simulink model "model_4_3_offset"  (R2020a)
settings: Solver=FixedStepAuto  StartTime=0.0  StopTime=10.0  FixedStep=0.002  RelTol=1e-3
settings Model: Creator=gianlu  LastModifiedBy=Shadman

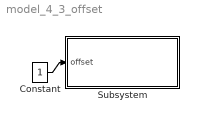
== system model_4_3_offset ==
  Constant : Constant
  Subsystem : Subsystem  StopFcn=|
      | % Cart dimensions
      | x_size = 0.2;
      | y_size = 0.05;
      | wheel_radius = 0.025
      | wheel_pos = 0.08
      | %%
      | % Cart body
      | x = [ - x_size, x_size, x_size, -x_size];
      | y = [ - y_size, -y_size, y_size, y_size];
      | 
      | %%
      | g = hgtransform;
      | %%
      | patch('XData',x,'YData',y,'FaceColor','red','Parent',g)
      | 
      | % Left wheel
      | theta = linspace(0, 2*pi, 15);
      | l_x = - wheel_pos + wheel_radius * cos(theta);
      | l_y = -(y_size + wheel_radius) + wheel_radius * sin(theta);
      | l = hgtransform;
      | patch('XData',l_x,'YData',l_y,'FaceColor','black','Parent', l)
      | 
      | 
      | % Right wheel
      | r_x = wheel_pos + wheel_radius*cos(theta);
      | r_y = -(y_size + wheel_radius) + wheel_radius*sin(theta);
      | r = hgtransform;
      | patch('XData',r_x,'YData',r_y,'FaceColor','black','Parent', r)
      | 
      | 
      | % Plot settings
      | axis equal
      | title('Cart animation')
      | set(gca,'YColor','none')
      | 
      | xlim([-1.5 1.5])
      | ylim([-(y_size+2*wheel_radius), 3 * y_size])
      | set(gca, 'Ytick', [])
      | pt1 = [0 0 0];
      | pt2 = [3 0 0];
      | %%
      | data_pos = out.sim_data_cart.signals.values(:,1);
      | tot_time_step=size(out.tout)/10;
      | 
      | %%
      | for i=1:1:tot_time_step(1)
      |   transf = makehgtform('translate', [1 0 0] * data_pos(i*5));
      |   set(g, 'Matrix', transf);
      |   set(l, 'Matrix', transf);
      |   set(r, 'Matrix', transf);
      | 
      |   %g.Matrix = makehgtform('translate', [1 0 0] * data_pos(i));
      |   %l.Matrix = makehgtform('translate', [1 0 0] * data_pos(i));
      |   %right.Matrix = makehgtform('translate', [1 0 0] * data_pos(i));
      |   %drawnow limitrate
      |   pause(0.02)
      | end
  wires:
  Constant/1 -> Subsystem/1("offset ")

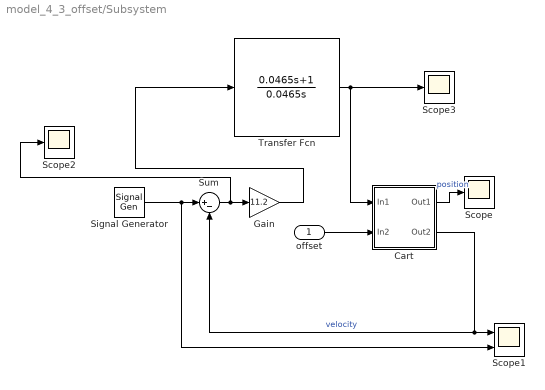
== system model_4_3_offset/Subsystem ==
  "offset " : Inport
  "Cart " : Subsystem  TreatAsAtomicUnit=on
  Gain : Gain  Gain=11.2
  Scope : Scope
  Scope1 : Scope  NumInputPorts=2
  Scope2 : Scope
  Scope3 : Scope
  Signal Generator : SignalGenerator  WaveForm=square  Amplitude=0.2  Frequency=0.5
  Sum : Sum  Inputs=|+-
  Transfer Fcn : TransferFcn  Numerator=[0.0465 1]  Denominator=[0.0465 0]
  wires:
  "offset "/1 -> "Cart "/2(In2)
  "Cart "/1(Out1) -> Scope/1  "position"
  "Cart "/2(Out2) -> Sum/2, Scope1/1  "velocity"
  Signal Generator/1 -> Scope1/2, Sum/1
  Transfer Fcn/1 -> Scope3/1, "Cart "/1(In1)
  Sum/1 -> Scope2/1, Gain/1
  Gain/1 -> Transfer Fcn/1

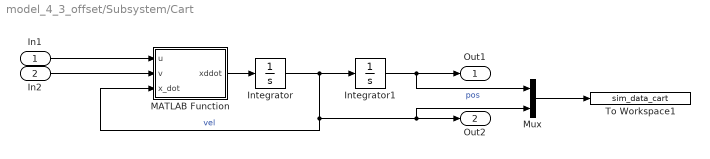
== system model_4_3_offset/Subsystem/Cart  ==
  In1 : Inport
  In2 : Inport  Port=2
  Integrator : Integrator
  Integrator1 : Integrator
  MATLAB Function : MATLAB Function  TreatAsAtomicUnit=on
  Mux : Mux  Inputs=2
  To Workspace1 : ToWorkspace  VariableName=sim_data_cart  SaveFormat=Structure With Time  SampleTime=-1
  Out1 : Outport
  Out2 : Outport  Port=2
  wires:
  MATLAB Function/1(xddot) -> Integrator/1
  Integrator/1 -> Mux/2, Out2/1, MATLAB Function/3(x_dot), Integrator1/1  "vel"
  In1/1 -> MATLAB Function/1(u)
  Integrator1/1 -> Mux/1, Out1/1  "pos"
  Mux/1 -> To Workspace1/1
  In2/1 -> MATLAB Function/2(v)

== matlab function model_4_3_offset/Subsystem/Cart /MATLAB Function ==
  data: u input; v input; xddot output; x_dot input
function xddot = fcn(u, v, x_dot)
% Dynamics settings. Check the accessory file []
alpha = 1.7189;
beta = 7.682;
M = 0.455;
% slope in radians
theta = 10 * pi / 180;
g = 9.81;
F = alpha * u - beta * x_dot;
% Friction coefficient 0.1 is chose arbitrarily (in a reasonable range anyway)
F_fric = -0.1 * x_dot;
xddot = (F + F_fric)/M + v * g * sin(theta);
